simulink model "test3channel_c"  (Simulink 7.1)
settings: Solver=VariableStepDiscrete  StartTime=0.0  StopTime=0.0  RelTol=1e-3
undefined symbols (not defined in the file): IScale
libraries: SaliencyLib x18
settings Model: Creator=bruce  LastModifiedBy=bruce

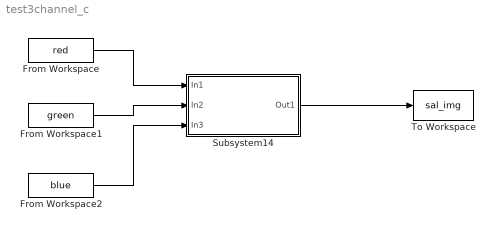
== system test3channel_c ==
  From Workspace : FromWorkspace  VariableName=red  SampleTime=0
  From Workspace1 : FromWorkspace  VariableName=green  SampleTime=0
  From Workspace2 : FromWorkspace  VariableName=blue  SampleTime=0
  Subsystem14 : Subsystem  AncestorBlock=SaliencyLib/Subsystem14  mask(Three Channel Saliency){inRows=256, inCols=256, sysxlr1=64, sysxlc1=64, sysxlr2=32, sysxlc2=32}
      mask prompts: inRows "input rows:"; inCols "input cols:"; sysxlr1 "x level rows 1"; sysxlc1 "x level cols 1"; sysxlr2 "x level rows 2"; sysxlc2 "x level cols 2"
      mask help:
      | Implements a three channel (intensity, orientation, color)
      | saliency map computaion based on the 1998 PAMI paper.
      mask Display:
      | fprintf('I-O-C CHANNEL\nSALIENCY\n(%s x %s)', get_param(gcb,'inRows'),get_param(gcb,'inCols'))
      | port_label('input',1,'r')
      | port_label('input',2,'g')
      | port_label('input',3,'b')
      | port_label('output',1,'SAL')
  To Workspace : ToWorkspace  VariableName=sal_img  SampleTime=-1  SaveFormat=Structure
  wires:
  From Workspace/1 -> Subsystem14/1(In1)
  From Workspace1/1 -> Subsystem14/2(In2)
  From Workspace2/1 -> Subsystem14/3(In3)
  Subsystem14/1(Out1) -> To Workspace/1

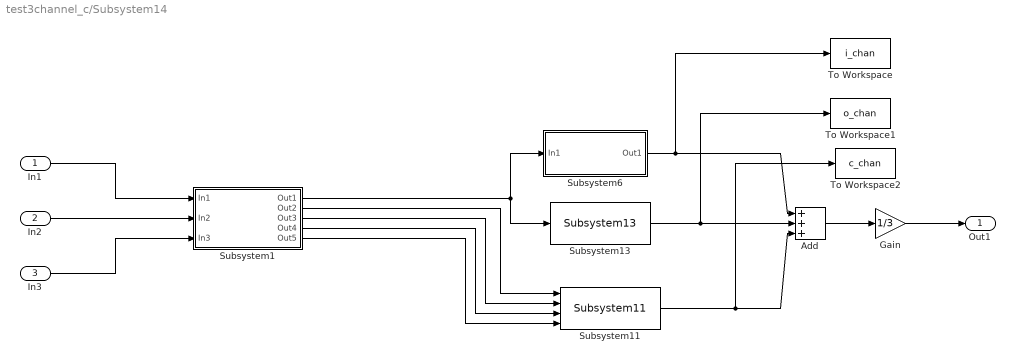
== system test3channel_c/Subsystem14 ==
  In1 : Inport  OutDataType=sfix(16)  OutScaling=2^0
  In2 : Inport  Port=2  OutDataType=sfix(16)  OutScaling=2^0
  In3 : Inport  Port=3  OutDataType=sfix(16)  OutScaling=2^0
  Add : Sum  Inputs=+++  OutDataType=sfix(16)  OutScaling=2^-10
  Gain : Gain  Gain=1/3  ParameterDataType=sfix(16)  ParameterScaling=2^0  OutDataType=sfix(16)  OutScaling=2^0
  Subsystem1 : Subsystem
      mask Display:
      | disp('COLOR\nMAPPING')
      | port_label('input',1,'r')
      | port_label('input',2','g')
      | port_label('input',3,'b')
      | port_label('output',1,'I')
      | port_label('output',2,'R')
      | port_label('output',3,'G')
      | port_label('output',4','B')
      | port_label('output',5,'Y')
  Subsystem11 : SaliencyLib/Subsystem11  SystemSampleTime=-1  br=inRows  bc=inCols
  Subsystem13 : SaliencyLib/Subsystem13  SystemSampleTime=-1  sr=inRows  sc=inCols
      link override Subsystem1: isr=sr  isc=sc
      link override Subsystem1/Subsystem7/Subsystem1: isr=inRows  isc=inCols
      link override Subsystem1/Subsystem7/Subsystem2: isr=inRows  isc=inCols
      link override Subsystem1/Subsystem7/Subsystem3: isr=inRows  isc=inCols
      link override Subsystem1/Subsystem7/Subsystem4: isr=inRows  isc=inCols
      link override Subsystem1/Subsystem7/Subsystem5: isr=inRows  isc=inCols
      link override Subsystem1/Subsystem7/Subsystem6: isr=inRows  isc=inCols
      link override Subsystem12: isr=sr  isc=sc
      link override Subsystem12/Subsystem7/Subsystem1: isr=inRows  isc=inCols
      link override Subsystem12/Subsystem7/Subsystem2: isr=inRows  isc=inCols
      link override Subsystem12/Subsystem7/Subsystem3: isr=inRows  isc=inCols
      link override Subsystem12/Subsystem7/Subsystem4: isr=inRows  isc=inCols
      link override Subsystem12/Subsystem7/Subsystem5: isr=inRows  isc=inCols
      link override Subsystem12/Subsystem7/Subsystem6: isr=inRows  isc=inCols
      link override Subsystem2: isr=sr  isc=sc
      link override Subsystem2/Subsystem7/Subsystem1: isr=inRows  isc=inCols
      link override Subsystem2/Subsystem7/Subsystem2: isr=inRows  isc=inCols
      link override Subsystem2/Subsystem7/Subsystem3: isr=inRows  isc=inCols
      link override Subsystem2/Subsystem7/Subsystem4: isr=inRows  isc=inCols
      link override Subsystem2/Subsystem7/Subsystem5: isr=inRows  isc=inCols
      link override Subsystem2/Subsystem7/Subsystem6: isr=inRows  isc=inCols
      link override Subsystem3: isr=sr  isc=sc
      link override Subsystem3/Subsystem7/Subsystem1: isr=inRows  isc=inCols
      link override Subsystem3/Subsystem7/Subsystem2: isr=inRows  isc=inCols
      link override Subsystem3/Subsystem7/Subsystem3: isr=inRows  isc=inCols
      link override Subsystem3/Subsystem7/Subsystem4: isr=inRows  isc=inCols
      link override Subsystem3/Subsystem7/Subsystem5: isr=inRows  isc=inCols
      link override Subsystem3/Subsystem7/Subsystem6: isr=inRows  isc=inCols
  Subsystem6 : Subsystem  AncestorBlock=SaliencyLib/Subsystem6  mask(Intensity Based Saliency Channel){isr=inRows, isc=inCols}
      mask prompts: isr "source rows:"; isc "source cols:"
      mask help:
      | Outputs a saliency map based on mulit-scale center-surround
      | intensity differences in the input image.
      mask Display: fprintf('INTENSITY CHANNEL\n(%s X %s)', get_param(gcb,'isr'),get_param(gcb,'isc'))
  To Workspace : ToWorkspace  VariableName=i_chan  SampleTime=-1  SaveFormat=Structure
  To Workspace1 : ToWorkspace  VariableName=o_chan  SampleTime=-1  SaveFormat=Structure
  To Workspace2 : ToWorkspace  VariableName=c_chan  SampleTime=-1  SaveFormat=Structure
  Out1 : Outport  OutDataType=sfix(16)  OutScaling=2^0
  wires:
  In1/1 -> Subsystem1/1(In1)
  Subsystem1/1(Out1) -> Subsystem6/1(In1), Subsystem13/1
  In2/1 -> Subsystem1/2(In2)
  In3/1 -> Subsystem1/3(In3)
  Subsystem1/2(Out2) -> Subsystem11/1
  Subsystem1/3(Out3) -> Subsystem11/2
  Subsystem1/4(Out4) -> Subsystem11/3
  Subsystem1/5(Out5) -> Subsystem11/4
  Subsystem11/1 -> Add/3, To Workspace2/1
  Subsystem6/1(Out1) -> Add/1, To Workspace/1
  Subsystem13/1 -> Add/2, To Workspace1/1
  Gain/1 -> Out1/1
  Add/1 -> Gain/1

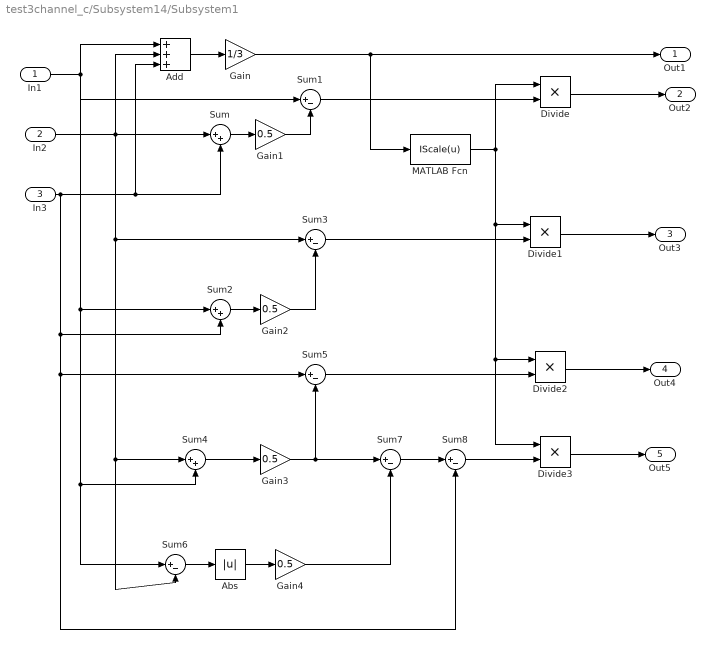
== system test3channel_c/Subsystem14/Subsystem1 ==
  In1 : Inport  OutDataType=sfix(16)  OutScaling=2^0
  In2 : Inport  Port=2  OutDataType=sfix(16)  OutScaling=2^0
  In3 : Inport  Port=3  OutDataType=sfix(16)  OutScaling=2^0
  Abs : Abs  OutDataType=sfix(16)  OutScaling=2^0
  Add : Sum  Inputs=+++  OutDataType=sfix(16)  OutScaling=2^-10
  Divide{,1..3} (4 alike) : Product  Inputs=**  OutDataType=sfix(16)  OutScaling=2^-10
  Gain : Gain  Gain=1/3  ParameterDataType=sfix(16)  ParameterScaling=2^0  OutDataType=sfix(16)  OutScaling=2^0
  Gain{1..4} (4 alike) : Gain  Gain=0.5  ParameterDataType=sfix(16)  ParameterScaling=2^0  OutDataType=sfix(16)  OutScaling=2^0
  MATLAB Fcn : MATLABFcn  MATLABFcn=IScale(u)  Output1D=off
  Sum : Sum  Inputs=|++  OutDataType=sfix(16)  OutScaling=2^0
  Sum{1,3,5..8} (6 alike) : Sum  Inputs=|+-  OutDataType=sfix(16)  OutScaling=2^0
  Sum2 : Sum  Inputs=|++  OutDataType=sfix(16)  OutScaling=2^0
  Sum4 : Sum  Inputs=|++  OutDataType=sfix(16)  OutScaling=2^0
  Out1 : Outport  OutDataType=sfix(16)  OutScaling=2^0
  Out2 : Outport  Port=2  OutDataType=sfix(16)  OutScaling=2^0
  Out3 : Outport  Port=3  OutDataType=sfix(16)  OutScaling=2^0
  Out4 : Outport  Port=4  OutDataType=sfix(16)  OutScaling=2^0
  Out5 : Outport  Port=5  OutDataType=sfix(16)  OutScaling=2^0
  wires:
  MATLAB Fcn/1 -> Divide3/1, Divide2/1, Divide1/1, Divide/1
  Divide3/1 -> Out5/1
  Sum8/1 -> Divide3/2
  Sum7/1 -> Sum8/1
  Gain4/1 -> Sum7/2
  Abs/1 -> Gain4/1
  Sum6/1 -> Abs/1
  Divide2/1 -> Out4/1
  Divide1/1 -> Out3/1
  Sum5/1 -> Divide2/2
  Sum3/1 -> Divide1/2
  Divide/1 -> Out2/1
  Sum1/1 -> Divide/2
  Sum4/1 -> Gain3/1
  Gain3/1 -> Sum7/1, Sum5/2
  Gain2/1 -> Sum3/2
  Sum2/1 -> Gain2/1
  Gain1/1 -> Sum1/2
  Sum/1 -> Gain1/1
  Add/1 -> Gain/1
  Gain/1 -> MATLAB Fcn/1, Out1/1
  In3/1 -> Sum8/2, Sum5/1, Sum2/2, Sum/2, Add/3
  In2/1 -> Sum6/2, Sum4/1, Sum3/1, Sum/1, Add/2
  In1/1 -> Sum6/1, Sum4/2, Sum2/1, Sum1/1, Add/1

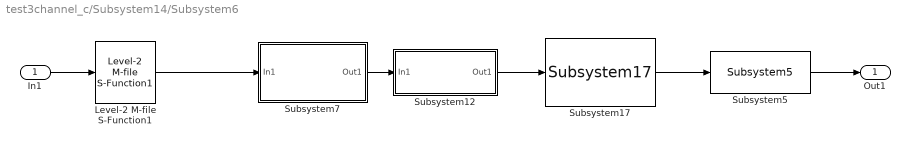
== system test3channel_c/Subsystem14/Subsystem6 ==
  In1 : Inport  OutDataType=sfix(16)  OutScaling=2^0
  Level-2 M-file S-Function1 : SaliencyLib/Level-2 M-file S-Function1  sr=isr  sc=isc  sl=8  bo=0
  Subsystem12 : Subsystem
      mask Display: disp('NORMALIZE')
  Subsystem17 : SaliencyLib/Subsystem17  SystemSampleTime=-1  brxs=isr  bcxs=isc  L1off=0  L2off=0
      link override Level-2 M-file S-Function: br=sysxlr1  bc=sysxlc1
      link override Level-2 M-file S-Function1: sr=sysxlr1  sc=sysxlc1
      link override Level-2 M-file S-Function2: sr=sysxlr1  sc=sysxlc1
      link override Level-2 M-file S-Function3: sr=sysxlr2  sc=sysxlc2
      link override Level-2 M-file S-Function4: sr=sysxlr2  sc=sysxlc2
      link override Level-2 M-file S-Function5: br=sysxlr1  bc=sysxlc1
      link override Level-2 M-file S-Function6: br=sysxlr2  bc=sysxlc2
      link override Level-2 M-file S-Function7: br=sysxlr2  bc=sysxlc2
  Subsystem5 : SaliencyLib/Subsystem5  SystemSampleTime=-1
  Subsystem7 : Subsystem
      mask Display:
      | disp('C/S\nCOMBINE')
      | port_label('input',1,'PYR')
      | port_label('output',1,'I-BUS')
  Out1 : Outport  OutDataType=sfix(16)  OutScaling=2^0
  wires:
  Subsystem12/1(Out1) -> Subsystem17/1
  Subsystem5/1 -> Out1/1
  Subsystem17/1 -> Subsystem5/1
  Subsystem7/1(Out1) -> Subsystem12/1(In1)
  Level-2 M-file S-Function1/1 -> Subsystem7/1(In1)
  In1/1 -> Level-2 M-file S-Function1/1

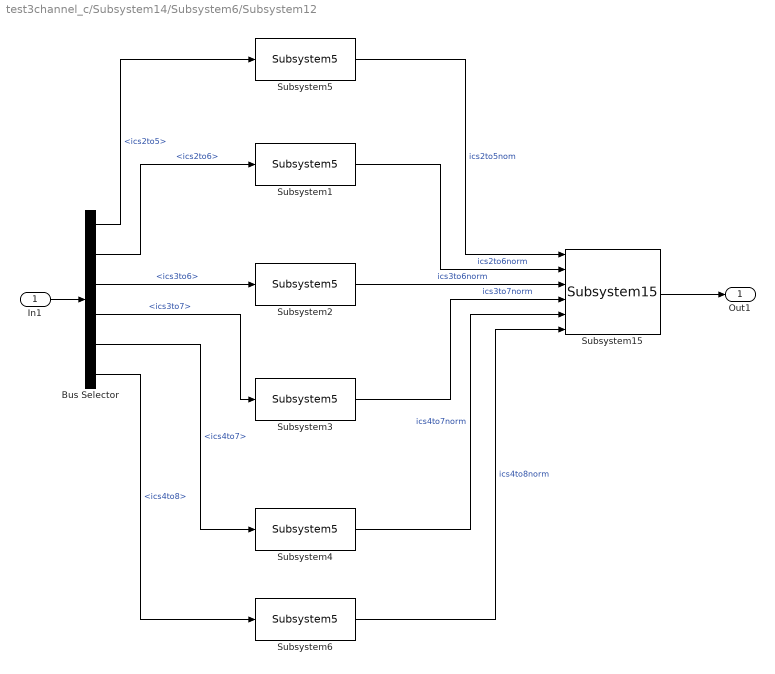
== system test3channel_c/Subsystem14/Subsystem6/Subsystem12 ==
  In1 : Inport  OutDataType=sfix(16)  OutScaling=2^0
  Bus Selector : BusSelector  OutputSignals=ics2to5,ics2to6,ics3to6,ics3to7,ics4to7,ics4to8
  Subsystem{1..6} (6 alike) : SaliencyLib/Subsystem5  SystemSampleTime=-1
  Subsystem15 : SaliencyLib/Subsystem15  SystemSampleTime=-1
  Out1 : Outport  OutDataType=sfix(16)  OutScaling=2^0
  wires:
  Subsystem15/1 -> Out1/1
  Subsystem6/1 -> Subsystem15/6  "ics4to8norm"
  Subsystem4/1 -> Subsystem15/5  "ics4to7norm"
  Subsystem3/1 -> Subsystem15/4  "ics3to7norm"
  Subsystem2/1 -> Subsystem15/3  "ics3to6norm"
  Subsystem1/1 -> Subsystem15/2  "ics2to6norm"
  Subsystem5/1 -> Subsystem15/1  "ics2to5nom"
  Bus Selector/6 -> Subsystem6/1  "<ics4to8>"
  Bus Selector/5 -> Subsystem4/1  "<ics4to7>"
  Bus Selector/4 -> Subsystem3/1  "<ics3to7>"
  Bus Selector/3 -> Subsystem2/1  "<ics3to6>"
  Bus Selector/2 -> Subsystem1/1  "<ics2to6>"
  Bus Selector/1 -> Subsystem5/1  "<ics2to5>"
  In1/1 -> Bus Selector/1

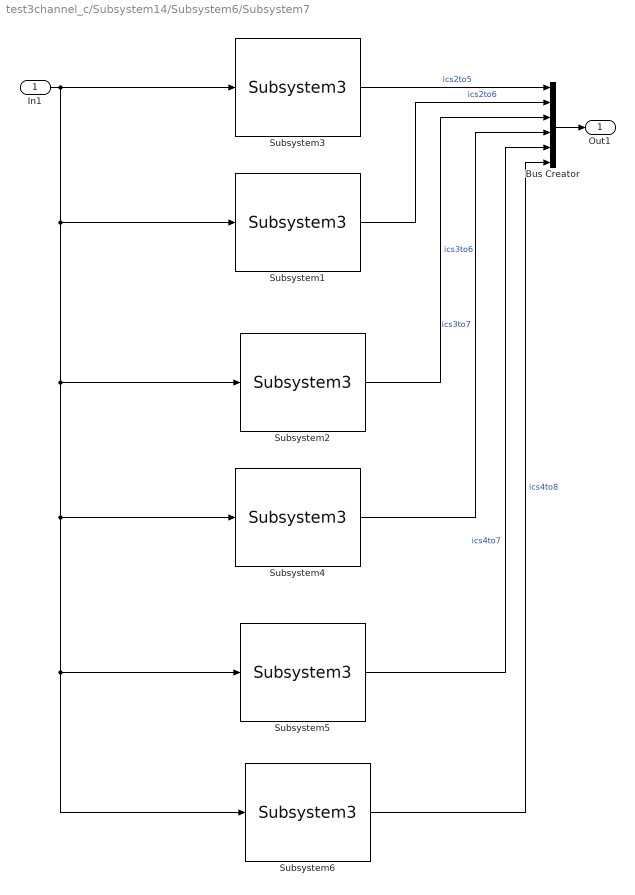
== system test3channel_c/Subsystem14/Subsystem6/Subsystem7 ==
  In1 : Inport  OutDataType=sfix(16)  OutScaling=2^0
  Bus Creator : BusCreator  Inputs=6
  Subsystem1 : SaliencyLib/Subsystem3  SystemSampleTime=-1  isr=isr  isc=isc
      link override Level-2 M-file S-Function1: Parameters=332,500,6  pl=6
      link override Level-2 M-file S-Function2: cl=6
  Subsystem2 : SaliencyLib/Subsystem3  SystemSampleTime=-1  isr=isr  isc=isc
      link override Level-2 M-file S-Function: Parameters=332,500,3  pl=3
      link override Level-2 M-file S-Function1: Parameters=332,500,6  pl=6
      link override Level-2 M-file S-Function2: fl=3  cl=6
  Subsystem3 : SaliencyLib/Subsystem3  SystemSampleTime=-1  isr=isr  isc=isc
      link override Level-2 M-file S-Function: br=isr  bc=isc
      link override Level-2 M-file S-Function1: Parameters=332,500,5
  Subsystem4 : SaliencyLib/Subsystem3  SystemSampleTime=-1  isr=isr  isc=isc
      link override Level-2 M-file S-Function: Parameters=332,500,3  pl=3
      link override Level-2 M-file S-Function1: Parameters=332,500,7  pl=7
      link override Level-2 M-file S-Function2: fl=3  cl=7
  Subsystem5 : SaliencyLib/Subsystem3  SystemSampleTime=-1  isr=isr  isc=isc
      link override Level-2 M-file S-Function: Parameters=332,500,4  pl=4
      link override Level-2 M-file S-Function1: Parameters=332,500,7  pl=7
      link override Level-2 M-file S-Function2: fl=4  cl=7
  Subsystem6 : SaliencyLib/Subsystem3  SystemSampleTime=-1  isr=isr  isc=isc
      link override Level-2 M-file S-Function: Parameters=332,500,4  pl=4
      link override Level-2 M-file S-Function1: Parameters=332,500,8  pl=8
      link override Level-2 M-file S-Function2: fl=4  cl=8
  Out1 : Outport  OutDataType=sfix(16)  OutScaling=2^0
  wires:
  Subsystem6/1 -> Bus Creator/6  "ics4to8"
  Subsystem5/1 -> Bus Creator/5  "ics4to7"
  Bus Creator/1 -> Out1/1
  Subsystem4/1 -> Bus Creator/4  "ics3to7"
  Subsystem3/1 -> Bus Creator/1  "ics2to5"
  Subsystem2/1 -> Bus Creator/3  "ics3to6"
  Subsystem1/1 -> Bus Creator/2  "ics2to6"
  In1/1 -> Subsystem3/1, Subsystem1/1, Subsystem6/1, Subsystem5/1, Subsystem4/1, Subsystem2/1
